simulink model "sampleModel7424_pp_1_1"  (R2018a)
settings: Solver=VariableStepAuto  StartTime=0.0  StopTime=10.0  RelTol=1e-3
undefined symbols (not defined in the file): DiscIntNeverNeededParam
libraries: simulink x211
(part 2 of 7)

== system sampleModel7424_pp_1_1/cfblk127 ==
  cfblk1 : Inport
  Action Port : ActionPort  ActionType=then
  cfblk10 : DiscreteFilter
  cfblk{5,7,9,11} (4 alike) : UnitDelay  SampleTime=-1
  cfblk12 : If  SampleTime=1
  cfblk18 : Subsystem  TreatAsAtomicUnit=on
  cfblk19 : Subsystem  TreatAsAtomicUnit=on
  cfblk20 : Delay
  cfblk21 : Delay
  cfblk3 : DiscreteIntegrator  SampleTime=-1  OutDataTypeStr=double  ICPrevOutput=DiscIntNeverNeededParam  ICPrevScaledInput=DiscIntNeverNeededParam
  cfblk4 : Delay
  cfblk6 : simulink/Continuous/PID Controller (2DOF)  Controller=PID  TimeDomain=Discrete-time  SampleTime=-1  IntegratorMethod=Forward Euler  FilterMethod=Forward Euler  Form=Parallel  UseFilter=on  ControllerParametersSource=internal  P=1  I=1  D=0  N=100  b=1  c=1  InitialConditionSource=internal  InitialConditionForIntegrator=0  InitialConditionForFilter=0  ExternalReset=none  LimitOutput=off  UpperSaturationLimit=inf  LowerSaturationLimit=-inf  LinearizeAsGain=off  AntiWindupMode=none  Kb=1  TrackingMode=off  Kt=1  PParamMin=[]  PParamMax=[]  IParamMin=[]  IParamMax=[]  DParamMin=[]  DParamMax=[]  NParamMin=[]  NParamMax=[]  bParamMin=[]  bParamMax=[]  cParamMin=[]  cParamMax=[]  KbParamMin=[]  KbParamMax=[]  KtParamMin=[]  KtParamMax=[]  POutMin=[]  POutMax=[]  IOutMin=[]  IOutMax=[]  DOutMin=[]  DOutMax=[]  NOutMin=[]  NOutMax=[]  bOutMin=[]  bOutMax=[]  cOutMin=[]  cOutMax=[]  KbOutMin=[]  KbOutMax=[]  KtOutMin=[]  KtOutMax=[]  IntegratorOutMin=[]  IntegratorOutMax=[]  FilterOutMin=[]  FilterOutMax=[]  SumOutMin=[]  SumOutMax=[]  Sum1OutMin=[]  Sum1OutMax=[]  Sum2OutMin=[]  Sum2OutMax=[]  Sum3OutMin=[]  Sum3OutMax=[]  SumI1OutMin=[]  SumI1OutMax=[]  SumI2OutMin=[]  SumI2OutMax=[]  SumI3OutMin=[]  SumI3OutMax=[]  SumDOutMin=[]  SumDOutMax=[]  SaturationOutMin=[]  SaturationOutMax=[]  IntegratorContinuousStateAttributes=''  IntegratorStateMustResolveToSignalObject=off  IntegratorRTWStateStorageClass=Auto  FilterContinuousStateAttributes=''  FilterStateMustResolveToSignalObject=off  FilterRTWStateStorageClass=Auto  DifferentiatorICPrevScaledInput=0  DifferentiatorOutMin=[]  DifferentiatorOutMax=[]  FilterDiffOutCoefMin=[]  FilterDiffOutCoefMax=[]  SumDenOutMin=[]  SumDenOutMax=[]  SumNumOutMin=[]  SumNumOutMax=[]  ReciprocalOutMin=[]  ReciprocalOutMax=[]  DivideOutMin=[]  DivideOutMax=[]  TunerSelectOption=Transfer Function Based (PID Tuner App)
  cfblk8 : simulink/Continuous/PID Controller  Controller=PID  TimeDomain=Discrete-time  SampleTime=-1  IntegratorMethod=Forward Euler  FilterMethod=Forward Euler  Form=Parallel  UseFilter=on  ControllerParametersSource=internal  P=1  I=1  D=0  N=100  InitialConditionSource=internal  InitialConditionForIntegrator=0  InitialConditionForFilter=0  ExternalReset=none  LimitOutput=off  UpperSaturationLimit=inf  LowerSaturationLimit=-inf  LinearizeAsGain=off  AntiWindupMode=none  Kb=1  TrackingMode=off  Kt=1  PParamMin=[]  PParamMax=[]  IParamMin=[]  IParamMax=[]  DParamMin=[]  DParamMax=[]  NParamMin=[]  NParamMax=[]  KbParamMin=[]  KbParamMax=[]  KtParamMin=[]  KtParamMax=[]  POutMin=[]  POutMax=[]  IOutMin=[]  IOutMax=[]  DOutMin=[]  DOutMax=[]  NOutMin=[]  NOutMax=[]  KbOutMin=[]  KbOutMax=[]  KtOutMin=[]  KtOutMax=[]  IntegratorOutMin=[]  IntegratorOutMax=[]  FilterOutMin=[]  FilterOutMax=[]  SumOutMin=[]  SumOutMax=[]  SumI1OutMin=[]  SumI1OutMax=[]  SumI2OutMin=[]  SumI2OutMax=[]  SumI3OutMin=[]  SumI3OutMax=[]  SumDOutMin=[]  SumDOutMax=[]  SaturationOutMin=[]  SaturationOutMax=[]  IntegratorContinuousStateAttributes=''  IntegratorStateMustResolveToSignalObject=off  IntegratorRTWStateStorageClass=Auto  FilterContinuousStateAttributes=''  FilterStateMustResolveToSignalObject=off  FilterRTWStateStorageClass=Auto  DifferentiatorICPrevScaledInput=0  DifferentiatorOutMin=[]  DifferentiatorOutMax=[]  FilterDiffOutCoefMin=[]  FilterDiffOutCoefMax=[]  SumDenOutMin=[]  SumDenOutMax=[]  SumNumOutMin=[]  SumNumOutMax=[]  ReciprocalOutMin=[]  ReciprocalOutMax=[]  DivideOutMin=[]  DivideOutMax=[]  TunerSelectOption=Transfer Function Based (PID Tuner App)
  cyemi_{227..230,239..240,253..262} (16 alike) : DataTypeConversion  OutDataTypeStr=double
  emi_{16,126,290,332} (4 alike) : UnaryMinus
  emi_127 : MATLAB Function  TreatAsAtomicUnit=on
  emi_17 : MATLAB Function  TreatAsAtomicUnit=on
  emi_291 : MATLAB Function  TreatAsAtomicUnit=on
  emi_333 : MATLAB Function  TreatAsAtomicUnit=on
  cfblk2 : Outport
  cfblk13 : Outport  Port=2
  cfblk14 : Outport  Port=3
  cfblk15 : Outport  Port=4
  cfblk16 : Outport  Port=5
  cfblk17 : Outport  Port=6
  wires:
  cfblk9/1 -> cfblk17/1
  cfblk8/1 -> cfblk2/1
  cfblk7/1 -> cyemi_253/1, cyemi_254/1
  cfblk19/1(cfblk2) -> cyemi_228/1, cyemi_257/1
  cfblk18/1(cfblk2) -> cyemi_255/1, cyemi_256/1
  cfblk10/1 -> cyemi_230/1, cyemi_258/1, cyemi_259/1
  cfblk6/1 -> cfblk16/1, cyemi_239/1, cyemi_261/1
  cfblk4/1 -> cfblk13/1
  cfblk1/1 -> cfblk14/1, cyemi_227/1
  cfblk3/1 -> cfblk15/1
  cfblk12/1 -> cfblk18/Action
  cfblk12/2 -> cfblk19/Action
  cyemi_227/1 -> cfblk10/1
  cyemi_228/1 -> cfblk11/1
  cyemi_229/1 -> cfblk12/1
  cfblk20/1 -> cyemi_229/1
  cyemi_230/1 -> cfblk18/1(cfblk1)
  cyemi_239/1 -> cfblk19/1(cfblk1)
  cyemi_240/1 -> cfblk19/2(cfblk10)
  cfblk21/1 -> cyemi_240/1
  cyemi_253/1 -> cfblk20/1, emi_126/1, emi_127/1(o)
  cyemi_254/1 -> cfblk21/1
  cyemi_255/1 -> cfblk3/1
  cyemi_256/1 -> cfblk4/1, emi_332/1, emi_333/1(o)
  cyemi_257/1 -> cfblk5/1, emi_290/1, emi_291/1(o)
  cyemi_258/1 -> cfblk6/1
  cyemi_259/1 -> cfblk6/2
  cyemi_260/1 -> cfblk7/1
  cfblk5/1 -> cyemi_260/1
  cyemi_261/1 -> cfblk8/1, emi_16/1, emi_17/1(o)
  cyemi_262/1 -> cfblk9/1
  cfblk11/1 -> cyemi_262/1
  emi_16/1 -> emi_17/2(e)
  emi_126/1 -> emi_127/2(e)
  emi_290/1 -> emi_291/2(e)
  emi_332/1 -> emi_333/2(e)

== system sampleModel7424_pp_1_1/cfblk128 ==
  cfblk1 : Inport
  cfblk9 : Inport  Port=2
  cfblk10 : Inport  Port=3
  Action Port : ActionPort  ActionType=else
  cfblk13 : DataTypeConversion  OutDataTypeStr=double
  cfblk14 : DataTypeConversion  OutDataTypeStr=double
  cfblk3 : simulink/Discrete/Transfer Fcn Lead or Lag  PoleZ=0.95  ZeroZ=0.75  ICPrevOutput=0.0  ICPrevInput=0.0  DoSatur=off
      settings: SourceProductName=Simulink  SourceProductBaseCode=SL
  cfblk4 : DiscreteIntegrator  SampleTime=-1  OutDataTypeStr=double  ICPrevOutput=DiscIntNeverNeededParam  ICPrevScaledInput=DiscIntNeverNeededParam
  cfblk5 : UnitDelay  SampleTime=-1
  cfblk6 : simulink/Discrete/Transfer Fcn First Order  PoleZ=0.95  ICPrevOutput=0.0  DoSatur=off
      settings: SourceProductName=Simulink
  cfblk7 : DiscreteStateSpace  SampleTime=-1
  cfblk8 : simulink/Discrete/Transfer Fcn Real Zero  ZeroZ=0.75  ICPrevInput=0.0  DoSatur=off
      settings: SourceProductName=Simulink  SourceProductBaseCode=SL
  cyemi_{266,269..270,272} (4 alike) : DataTypeConversion  OutDataTypeStr=double
  cyemi_267 : DataTypeConversion  OutDataTypeStr=fixdt('ufix16_E3')
  cyemi_268 : DataTypeConversion  OutDataTypeStr=uint16
  cyemi_271 : DataTypeConversion  OutDataTypeStr=fixdt('ufix16_E3')
  cyemi_273 : DataTypeConversion  OutDataTypeStr=fixdt('ufix16_E3')
  cfblk2 : Outport
  cfblk11 : Outport  Port=2
  cfblk12 : Outport  Port=3
  wires:
  cfblk5/1 -> cfblk11/1
  cfblk7/1 -> cfblk12/1
  cfblk10/1 -> cfblk2/1
  cyemi_266/1 -> cfblk13/1
  cfblk4/1 -> cyemi_266/1
  cyemi_267/1 -> cfblk14/1
  cfblk6/1 -> cyemi_267/1
  cyemi_268/1 -> cfblk3/1
  cfblk1/1 -> cyemi_268/1
  cyemi_269/1 -> cfblk4/1
  cfblk14/1 -> cyemi_269/1
  cyemi_270/1 -> cfblk5/1
  cfblk9/1 -> cyemi_270/1
  cyemi_271/1 -> cfblk6/1
  cfblk8/1 -> cyemi_271/1
  cyemi_272/1 -> cfblk7/1
  cfblk13/1 -> cyemi_272/1
  cyemi_273/1 -> cfblk8/1
  cfblk3/1 -> cyemi_273/1

== system sampleModel7424_pp_1_1/cfblk129 ==
  cfblk1 : Inport
  cfblk8 : Inport  Port=2
  Action Port : ActionPort  ActionType=then
  cfblk10 : Delay
  cfblk3 : UnitDelay  SampleTime=-1
  cfblk4 : simulink/Continuous/PID Controller (2DOF)  Controller=PID  TimeDomain=Discrete-time  SampleTime=-1  IntegratorMethod=Forward Euler  FilterMethod=Forward Euler  Form=Parallel  UseFilter=on  ControllerParametersSource=internal  P=1  I=1  D=0  N=100  b=1  c=1  InitialConditionSource=internal  InitialConditionForIntegrator=0  InitialConditionForFilter=0  ExternalReset=none  LimitOutput=off  UpperSaturationLimit=inf  LowerSaturationLimit=-inf  LinearizeAsGain=off  AntiWindupMode=none  Kb=1  TrackingMode=off  Kt=1  PParamMin=[]  PParamMax=[]  IParamMin=[]  IParamMax=[]  DParamMin=[]  DParamMax=[]  NParamMin=[]  NParamMax=[]  bParamMin=[]  bParamMax=[]  cParamMin=[]  cParamMax=[]  KbParamMin=[]  KbParamMax=[]  KtParamMin=[]  KtParamMax=[]  POutMin=[]  POutMax=[]  IOutMin=[]  IOutMax=[]  DOutMin=[]  DOutMax=[]  NOutMin=[]  NOutMax=[]  bOutMin=[]  bOutMax=[]  cOutMin=[]  cOutMax=[]  KbOutMin=[]  KbOutMax=[]  KtOutMin=[]  KtOutMax=[]  IntegratorOutMin=[]  IntegratorOutMax=[]  FilterOutMin=[]  FilterOutMax=[]  SumOutMin=[]  SumOutMax=[]  Sum1OutMin=[]  Sum1OutMax=[]  Sum2OutMin=[]  Sum2OutMax=[]  Sum3OutMin=[]  Sum3OutMax=[]  SumI1OutMin=[]  SumI1OutMax=[]  SumI2OutMin=[]  SumI2OutMax=[]  SumI3OutMin=[]  SumI3OutMax=[]  SumDOutMin=[]  SumDOutMax=[]  SaturationOutMin=[]  SaturationOutMax=[]  IntegratorContinuousStateAttributes=''  IntegratorStateMustResolveToSignalObject=off  IntegratorRTWStateStorageClass=Auto  FilterContinuousStateAttributes=''  FilterStateMustResolveToSignalObject=off  FilterRTWStateStorageClass=Auto  DifferentiatorICPrevScaledInput=0  DifferentiatorOutMin=[]  DifferentiatorOutMax=[]  FilterDiffOutCoefMin=[]  FilterDiffOutCoefMax=[]  SumDenOutMin=[]  SumDenOutMax=[]  SumNumOutMin=[]  SumNumOutMax=[]  ReciprocalOutMin=[]  ReciprocalOutMax=[]  DivideOutMin=[]  DivideOutMax=[]  TunerSelectOption=Transfer Function Based (PID Tuner App)
  cfblk5 : simulink/Continuous/PID Controller (2DOF)  Controller=PID  TimeDomain=Discrete-time  SampleTime=-1  IntegratorMethod=Forward Euler  FilterMethod=Forward Euler  Form=Parallel  UseFilter=on  ControllerParametersSource=internal  P=1  I=1  D=0  N=100  b=1  c=1  InitialConditionSource=internal  InitialConditionForIntegrator=0  InitialConditionForFilter=0  ExternalReset=none  LimitOutput=off  UpperSaturationLimit=inf  LowerSaturationLimit=-inf  LinearizeAsGain=off  AntiWindupMode=none  Kb=1  TrackingMode=off  Kt=1  PParamMin=[]  PParamMax=[]  IParamMin=[]  IParamMax=[]  DParamMin=[]  DParamMax=[]  NParamMin=[]  NParamMax=[]  bParamMin=[]  bParamMax=[]  cParamMin=[]  cParamMax=[]  KbParamMin=[]  KbParamMax=[]  KtParamMin=[]  KtParamMax=[]  POutMin=[]  POutMax=[]  IOutMin=[]  IOutMax=[]  DOutMin=[]  DOutMax=[]  NOutMin=[]  NOutMax=[]  bOutMin=[]  bOutMax=[]  cOutMin=[]  cOutMax=[]  KbOutMin=[]  KbOutMax=[]  KtOutMin=[]  KtOutMax=[]  IntegratorOutMin=[]  IntegratorOutMax=[]  FilterOutMin=[]  FilterOutMax=[]  SumOutMin=[]  SumOutMax=[]  Sum1OutMin=[]  Sum1OutMax=[]  Sum2OutMin=[]  Sum2OutMax=[]  Sum3OutMin=[]  Sum3OutMax=[]  SumI1OutMin=[]  SumI1OutMax=[]  SumI2OutMin=[]  SumI2OutMax=[]  SumI3OutMin=[]  SumI3OutMax=[]  SumDOutMin=[]  SumDOutMax=[]  SaturationOutMin=[]  SaturationOutMax=[]  IntegratorContinuousStateAttributes=''  IntegratorStateMustResolveToSignalObject=off  IntegratorRTWStateStorageClass=Auto  FilterContinuousStateAttributes=''  FilterStateMustResolveToSignalObject=off  FilterRTWStateStorageClass=Auto  DifferentiatorICPrevScaledInput=0  DifferentiatorOutMin=[]  DifferentiatorOutMax=[]  FilterDiffOutCoefMin=[]  FilterDiffOutCoefMax=[]  SumDenOutMin=[]  SumDenOutMax=[]  SumNumOutMin=[]  SumNumOutMax=[]  ReciprocalOutMin=[]  ReciprocalOutMax=[]  DivideOutMin=[]  DivideOutMax=[]  TunerSelectOption=Transfer Function Based (PID Tuner App)
  cfblk6 : UnitDelay  SampleTime=-1
  cfblk7 : simulink/Discrete/Transfer Fcn Lead or Lag  PoleZ=0.95  ZeroZ=0.75  ICPrevOutput=0.0  ICPrevInput=0.0  DoSatur=off
      settings: SourceProductName=Simulink  SourceProductBaseCode=SL
  cyemi_{276..283} (8 alike) : DataTypeConversion  OutDataTypeStr=double
  cfblk2 : Outport
  cfblk9 : Outport  Port=2
  wires:
  cfblk7/1 -> cfblk9/1
  cfblk8/1 -> cfblk2/1, cyemi_277/1, cyemi_281/1
  cyemi_276/1 -> cfblk10/1
  cfblk5/1 -> cyemi_276/1
  cyemi_277/1 -> cfblk3/1
  cyemi_278/1 -> cfblk4/1
  cfblk3/1 -> cyemi_278/1
  cyemi_279/1 -> cfblk4/2
  cfblk10/1 -> cyemi_279/1
  cyemi_280/1 -> cfblk5/1
  cfblk6/1 -> cyemi_280/1
  cyemi_281/1 -> cfblk5/2
  cyemi_282/1 -> cfblk6/1
  cfblk4/1 -> cyemi_282/1
  cyemi_283/1 -> cfblk7/1
  cfblk1/1 -> cyemi_283/1

== system sampleModel7424_pp_1_1/cfblk130 ==
  cfblk1 : Inport
  cfblk7 : Inport  Port=2
  cfblk8 : Inport  Port=3
  Action Port : ActionPort  ActionType=else
  cfblk11 : Subsystem  TreatAsAtomicUnit=on
  cfblk12 : Subsystem  TreatAsAtomicUnit=on
  cfblk13 : Delay
  cfblk14 : Delay
  cfblk3 : DiscreteFir
  cfblk4 : simulink/Continuous/PID Controller  Controller=PID  TimeDomain=Discrete-time  SampleTime=-1  IntegratorMethod=Forward Euler  FilterMethod=Forward Euler  Form=Parallel  UseFilter=on  ControllerParametersSource=internal  P=1  I=1  D=0  N=100  InitialConditionSource=internal  InitialConditionForIntegrator=0  InitialConditionForFilter=0  ExternalReset=none  LimitOutput=off  UpperSaturationLimit=inf  LowerSaturationLimit=-inf  LinearizeAsGain=off  AntiWindupMode=none  Kb=1  TrackingMode=off  Kt=1  PParamMin=[]  PParamMax=[]  IParamMin=[]  IParamMax=[]  DParamMin=[]  DParamMax=[]  NParamMin=[]  NParamMax=[]  KbParamMin=[]  KbParamMax=[]  KtParamMin=[]  KtParamMax=[]  POutMin=[]  POutMax=[]  IOutMin=[]  IOutMax=[]  DOutMin=[]  DOutMax=[]  NOutMin=[]  NOutMax=[]  KbOutMin=[]  KbOutMax=[]  KtOutMin=[]  KtOutMax=[]  IntegratorOutMin=[]  IntegratorOutMax=[]  FilterOutMin=[]  FilterOutMax=[]  SumOutMin=[]  SumOutMax=[]  SumI1OutMin=[]  SumI1OutMax=[]  SumI2OutMin=[]  SumI2OutMax=[]  SumI3OutMin=[]  SumI3OutMax=[]  SumDOutMin=[]  SumDOutMax=[]  SaturationOutMin=[]  SaturationOutMax=[]  IntegratorContinuousStateAttributes=''  IntegratorStateMustResolveToSignalObject=off  IntegratorRTWStateStorageClass=Auto  FilterContinuousStateAttributes=''  FilterStateMustResolveToSignalObject=off  FilterRTWStateStorageClass=Auto  DifferentiatorICPrevScaledInput=0  DifferentiatorOutMin=[]  DifferentiatorOutMax=[]  FilterDiffOutCoefMin=[]  FilterDiffOutCoefMax=[]  SumDenOutMin=[]  SumDenOutMax=[]  SumNumOutMin=[]  SumNumOutMax=[]  ReciprocalOutMin=[]  ReciprocalOutMax=[]  DivideOutMin=[]  DivideOutMax=[]  TunerSelectOption=Transfer Function Based (PID Tuner App)
  cfblk5 : UnitDelay  SampleTime=-1
  cfblk6 : If  SampleTime=1
  cyemi_{288..289,299..302,315..319} (11 alike) : DataTypeConversion  OutDataTypeStr=double
  cyemi_303 : DataTypeConversion  OutDataTypeStr=uint32
  cyemi_320 : DataTypeConversion  OutDataTypeStr=uint32
  emi_338 : UnaryMinus
  emi_339 : MATLAB Function  TreatAsAtomicUnit=on
  emi_50 : UnaryMinus
  emi_51 : MATLAB Function  TreatAsAtomicUnit=on
  cfblk2 : Outport
  cfblk9 : Outport  Port=2
  cfblk10 : Outport  Port=3
  wires:
  cfblk1/1 -> cyemi_288/1, cyemi_301/1
  cfblk11/2(cfblk10) -> cfblk2/1
  cfblk11/3(cfblk11) -> cfblk9/1, cyemi_302/1
  cfblk8/1 -> cyemi_303/1, cyemi_320/1
  cfblk12/1(cfblk2) -> cfblk10/1
  cfblk6/1 -> cfblk11/Action
  cfblk6/2 -> cfblk12/Action
  cyemi_288/1 -> cfblk11/1(cfblk1)
  cyemi_289/1 -> cfblk11/2(cfblk9)
  cfblk14/1 -> cyemi_289/1
  cyemi_299/1 -> cfblk12/1(cfblk1)
  cfblk13/1 -> cyemi_299/1
  cyemi_300/1 -> cfblk12/2(cfblk13)
  cfblk4/1 -> cyemi_300/1
  cyemi_301/1 -> cfblk12/3(cfblk14)
  cyemi_302/1 -> cfblk12/4(cfblk15)
  cyemi_303/1 -> cfblk12/5(cfblk16)
  cyemi_315/1 -> cfblk13/1, emi_338/1, emi_339/1(o)
  cfblk5/1 -> cyemi_315/1
  cyemi_316/1 -> cfblk14/1
  cfblk12/2(cfblk17) -> cyemi_316/1
  cyemi_317/1 -> cfblk3/1
  cfblk11/1(cfblk2) -> cyemi_317/1
  cyemi_318/1 -> cfblk4/1, emi_50/1, emi_51/1(o)
  cfblk7/1 -> cyemi_318/1
  cyemi_319/1 -> cfblk5/1
  cfblk3/1 -> cyemi_319/1
  cyemi_320/1 -> cfblk6/1
  emi_50/1 -> emi_51/2(e)
  emi_338/1 -> emi_339/2(e)

== system sampleModel7424_pp_1_1/cfblk131 ==
  cfblk1 : Inport
  cfblk13 : Inport  Port=2
  cfblk14 : Inport  Port=3
  Action Port : ActionPort  ActionType=then
  cfblk10 : simulink/Discrete/Transfer Fcn First Order  PoleZ=0.95  ICPrevOutput=0.0  DoSatur=off
      settings: SourceProductName=Simulink
  cfblk11 : simulink/Discrete/Difference  ICPrevInput=0.0  OutMin=[]  OutMax=[]  OutDataTypeStr=double  OutputDataTypeScalingMode=double  OutDataType=fixdt(1, 16)  OutScaling=2^-10  DoSatur=off
  cfblk12 : If  SampleTime=1
  cfblk16 : Subsystem  TreatAsAtomicUnit=on
  cfblk17 : Subsystem  TreatAsAtomicUnit=on
  cfblk{8,18..20} (4 alike) : Delay
  cfblk3 : simulink/Discrete/Tapped Delay  vinit=0.0  samptime=-1  NumDelays=1  DelayOrder=Oldest  includeCurrent=off
  cfblk4 : DiscreteStateSpace  SampleTime=-1
  cfblk5 : Delay  DelayLengthSource=Input port
      settings: InputPortMap=u0,p1
  cfblk6 : Delay  ShowEnablePort=on
      settings: InputPortMap=u0,e6
  cfblk7 : simulink/Discrete/Transfer Fcn First Order  PoleZ=0.95  ICPrevOutput=0.0  DoSatur=off
      settings: SourceProductName=Simulink
  cfblk9 : DiscreteIntegrator  SampleTime=-1  OutDataTypeStr=double  ICPrevOutput=DiscIntNeverNeededParam  ICPrevScaledInput=DiscIntNeverNeededParam
  cyemi_{324..328,340..341,347..358} (19 alike) : DataTypeConversion  OutDataTypeStr=double
  cfblk2 : Outport
  cfblk15 : Outport  Port=2
  wires:
  cfblk9/1 -> cfblk2/1, cyemi_354/1
  cfblk17/1(cfblk2) -> cyemi_325/1, cyemi_352/1
  cfblk8/1 -> cfblk15/1, cyemi_353/1
  cfblk12/1 -> cfblk16/Action
  cfblk12/2 -> cfblk17/Action
  cyemi_324/1 -> cfblk10/1
  cfblk16/2(cfblk13) -> cyemi_324/1
  cyemi_325/1 -> cfblk11/1
  cyemi_326/1 -> cfblk12/1
  cfblk14/1 -> cyemi_326/1
  cyemi_327/1 -> cfblk16/1(cfblk1)
  cfblk18/1 -> cyemi_327/1
  cyemi_328/1 -> cfblk16/2(cfblk12)
  cfblk3/1 -> cyemi_328/1
  cyemi_340/1 -> cfblk17/1(cfblk1)
  cfblk19/1 -> cyemi_340/1
  cyemi_341/1 -> cfblk17/2(cfblk8)
  cfblk20/1 -> cyemi_341/1
  cyemi_347/1 -> cfblk18/1
  cfblk5/1 -> cyemi_347/1
  cyemi_348/1 -> cfblk19/1
  cfblk4/1 -> cyemi_348/1
  cyemi_349/1 -> cfblk20/1
  cfblk11/1 -> cyemi_349/1
  cyemi_350/1 -> cfblk3/1
  cfblk1/1 -> cyemi_350/1
  cyemi_351/1 -> cfblk4/1
  cfblk10/1 -> cyemi_351/1
  cyemi_352/1 -> cfblk5/1
  cyemi_353/1 -> cfblk5/2
  cyemi_354/1 -> cfblk6/1
  cyemi_355/1 -> cfblk6/2
  cfblk7/1 -> cyemi_355/1
  cyemi_356/1 -> cfblk7/1
  cfblk13/1 -> cyemi_356/1
  cyemi_357/1 -> cfblk8/1
  cfblk6/1 -> cyemi_357/1
  cyemi_358/1 -> cfblk9/1
  cfblk16/1(cfblk2) -> cyemi_358/1

== system sampleModel7424_pp_1_1/cfblk132 ==
  cfblk1 : Inport
  cfblk13 : Inport  Port=2
  cfblk14 : Inport  Port=3
  Action Port : ActionPort  ActionType=else
  cfblk10 : simulink/Continuous/PID Controller (2DOF)  Controller=PID  TimeDomain=Discrete-time  SampleTime=-1  IntegratorMethod=Forward Euler  FilterMethod=Forward Euler  Form=Parallel  UseFilter=on  ControllerParametersSource=internal  P=1  I=1  D=0  N=100  b=1  c=1  InitialConditionSource=internal  InitialConditionForIntegrator=0  InitialConditionForFilter=0  ExternalReset=none  LimitOutput=off  UpperSaturationLimit=inf  LowerSaturationLimit=-inf  LinearizeAsGain=off  AntiWindupMode=none  Kb=1  TrackingMode=off  Kt=1  PParamMin=[]  PParamMax=[]  IParamMin=[]  IParamMax=[]  DParamMin=[]  DParamMax=[]  NParamMin=[]  NParamMax=[]  bParamMin=[]  bParamMax=[]  cParamMin=[]  cParamMax=[]  KbParamMin=[]  KbParamMax=[]  KtParamMin=[]  KtParamMax=[]  POutMin=[]  POutMax=[]  IOutMin=[]  IOutMax=[]  DOutMin=[]  DOutMax=[]  NOutMin=[]  NOutMax=[]  bOutMin=[]  bOutMax=[]  cOutMin=[]  cOutMax=[]  KbOutMin=[]  KbOutMax=[]  KtOutMin=[]  KtOutMax=[]  IntegratorOutMin=[]  IntegratorOutMax=[]  FilterOutMin=[]  FilterOutMax=[]  SumOutMin=[]  SumOutMax=[]  Sum1OutMin=[]  Sum1OutMax=[]  Sum2OutMin=[]  Sum2OutMax=[]  Sum3OutMin=[]  Sum3OutMax=[]  SumI1OutMin=[]  SumI1OutMax=[]  SumI2OutMin=[]  SumI2OutMax=[]  SumI3OutMin=[]  SumI3OutMax=[]  SumDOutMin=[]  SumDOutMax=[]  SaturationOutMin=[]  SaturationOutMax=[]  IntegratorContinuousStateAttributes=''  IntegratorStateMustResolveToSignalObject=off  IntegratorRTWStateStorageClass=Auto  FilterContinuousStateAttributes=''  FilterStateMustResolveToSignalObject=off  FilterRTWStateStorageClass=Auto  DifferentiatorICPrevScaledInput=0  DifferentiatorOutMin=[]  DifferentiatorOutMax=[]  FilterDiffOutCoefMin=[]  FilterDiffOutCoefMax=[]  SumDenOutMin=[]  SumDenOutMax=[]  SumNumOutMin=[]  SumNumOutMax=[]  ReciprocalOutMin=[]  ReciprocalOutMax=[]  DivideOutMin=[]  DivideOutMax=[]  TunerSelectOption=Transfer Function Based (PID Tuner App)
  cfblk11 : Delay
  cfblk12 : DiscreteFilter
  cfblk15 : Delay
  cfblk3 : simulink/Discrete/Transfer Fcn Real Zero  ZeroZ=0.75  ICPrevInput=0.0  DoSatur=off
      settings: SourceProductName=Simulink  SourceProductBaseCode=SL
  cfblk4 : DiscreteFir
  cfblk5 : DiscreteFilter
  cfblk6 : DiscreteIntegrator  SampleTime=-1  OutDataTypeStr=double  ICPrevOutput=DiscIntNeverNeededParam  ICPrevScaledInput=DiscIntNeverNeededParam
  cfblk7 : Delay  ShowEnablePort=on
      settings: InputPortMap=u0,e6
  cfblk8 : Delay  DelayLengthSource=Input port
      settings: InputPortMap=u0,p1
  cfblk9 : simulink/Discrete/Transfer Fcn First Order  PoleZ=0.95  ICPrevOutput=0.0  DoSatur=off
      settings: SourceProductName=Simulink
  cyemi_{362..363,365..375} (13 alike) : DataTypeConversion  OutDataTypeStr=double
  cyemi_364 : DataTypeConversion  OutDataTypeStr=uint16
  emi_{42,62,134,138,198} (5 alike) : UnaryMinus
  emi_135 : MATLAB Function  TreatAsAtomicUnit=on
  emi_139 : MATLAB Function  TreatAsAtomicUnit=on
  emi_199 : MATLAB Function  TreatAsAtomicUnit=on
  emi_43 : MATLAB Function  TreatAsAtomicUnit=on
  emi_63 : MATLAB Function  TreatAsAtomicUnit=on
  cfblk2 : Outport
  wires:
  cfblk13/1 -> cyemi_368/1, cyemi_375/1
  cfblk11/1 -> cfblk2/1
  cyemi_362/1 -> cfblk10/1, emi_198/1, emi_199/1(o)
  cfblk4/1 -> cyemi_362/1
  cyemi_363/1 -> cfblk10/2
  cfblk5/1 -> cyemi_363/1
  cyemi_364/1 -> cfblk11/1
  cfblk14/1 -> cyemi_364/1
  cyemi_365/1 -> cfblk12/1, emi_62/1, emi_63/1(o), emi_134/1, emi_135/1(o)
  cfblk6/1 -> cyemi_365/1
  cyemi_366/1 -> cfblk15/1, emi_138/1, emi_139/1(o)
  cfblk3/1 -> cyemi_366/1
  cyemi_367/1 -> cfblk3/1
  cfblk7/1 -> cyemi_367/1
  cyemi_368/1 -> cfblk4/1
  cyemi_369/1 -> cfblk5/1, emi_42/1, emi_43/1(o)
  cfblk1/1 -> cyemi_369/1
  cyemi_370/1 -> cfblk6/1
  cfblk9/1 -> cyemi_370/1
  cyemi_371/1 -> cfblk7/1
  cfblk8/1 -> cyemi_371/1
  cyemi_372/1 -> cfblk7/2
  cfblk12/1 -> cyemi_372/1
  cyemi_373/1 -> cfblk8/1
  cfblk15/1 -> cyemi_373/1
  cyemi_374/1 -> cfblk8/2
  cfblk10/1 -> cyemi_374/1
  cyemi_375/1 -> cfblk9/1
  emi_42/1 -> emi_43/2(e)
  emi_62/1 -> emi_63/2(e)
  emi_134/1 -> emi_135/2(e)
  emi_138/1 -> emi_139/2(e)
  emi_198/1 -> emi_199/2(e)

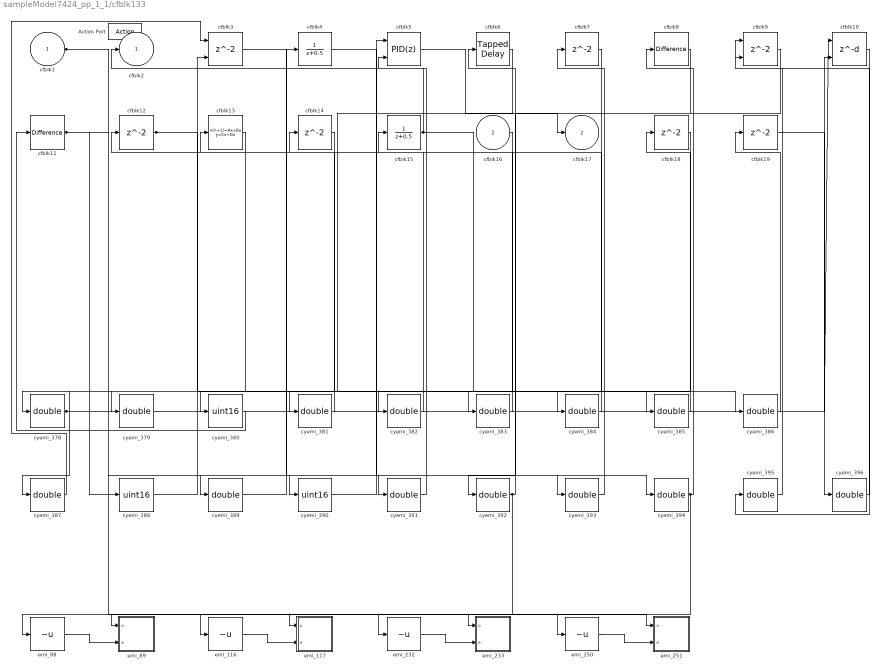
== system sampleModel7424_pp_1_1/cfblk133 ==
  cfblk1 : Inport
  cfblk16 : Inport  Port=2
  Action Port : ActionPort  ActionType=then
  cfblk10 : Delay  DelayLengthSource=Input port
      settings: InputPortMap=u0,p1
  cfblk11 : simulink/Discrete/Difference  ICPrevInput=0.0  OutMin=[]  OutMax=[]  OutDataTypeStr=uint16  OutputDataTypeScalingMode=uint16  OutDataType=fixdt(1, 16)  OutScaling=2^-10  DoSatur=off
  cfblk{7,12,14,18..19} (5 alike) : Delay
  cfblk13 : DiscreteStateSpace  SampleTime=-1
  cfblk15 : DiscreteTransferFcn
  cfblk3 : Delay  ShowEnablePort=on
      settings: InputPortMap=u0,e6
  cfblk4 : DiscreteTransferFcn
  cfblk5 : simulink/Continuous/PID Controller (2DOF)  Controller=PID  TimeDomain=Discrete-time  SampleTime=-1  IntegratorMethod=Forward Euler  FilterMethod=Forward Euler  Form=Parallel  UseFilter=on  ControllerParametersSource=internal  P=1  I=1  D=0  N=100  b=1  c=1  InitialConditionSource=internal  InitialConditionForIntegrator=0  InitialConditionForFilter=0  ExternalReset=none  LimitOutput=off  UpperSaturationLimit=inf  LowerSaturationLimit=-inf  LinearizeAsGain=off  AntiWindupMode=none  Kb=1  TrackingMode=off  Kt=1  PParamMin=[]  PParamMax=[]  IParamMin=[]  IParamMax=[]  DParamMin=[]  DParamMax=[]  NParamMin=[]  NParamMax=[]  bParamMin=[]  bParamMax=[]  cParamMin=[]  cParamMax=[]  KbParamMin=[]  KbParamMax=[]  KtParamMin=[]  KtParamMax=[]  POutMin=[]  POutMax=[]  IOutMin=[]  IOutMax=[]  DOutMin=[]  DOutMax=[]  NOutMin=[]  NOutMax=[]  bOutMin=[]  bOutMax=[]  cOutMin=[]  cOutMax=[]  KbOutMin=[]  KbOutMax=[]  KtOutMin=[]  KtOutMax=[]  IntegratorOutMin=[]  IntegratorOutMax=[]  FilterOutMin=[]  FilterOutMax=[]  SumOutMin=[]  SumOutMax=[]  Sum1OutMin=[]  Sum1OutMax=[]  Sum2OutMin=[]  Sum2OutMax=[]  Sum3OutMin=[]  Sum3OutMax=[]  SumI1OutMin=[]  SumI1OutMax=[]  SumI2OutMin=[]  SumI2OutMax=[]  SumI3OutMin=[]  SumI3OutMax=[]  SumDOutMin=[]  SumDOutMax=[]  SaturationOutMin=[]  SaturationOutMax=[]  IntegratorContinuousStateAttributes=''  IntegratorStateMustResolveToSignalObject=off  IntegratorRTWStateStorageClass=Auto  FilterContinuousStateAttributes=''  FilterStateMustResolveToSignalObject=off  FilterRTWStateStorageClass=Auto  DifferentiatorICPrevScaledInput=0  DifferentiatorOutMin=[]  DifferentiatorOutMax=[]  FilterDiffOutCoefMin=[]  FilterDiffOutCoefMax=[]  SumDenOutMin=[]  SumDenOutMax=[]  SumNumOutMin=[]  SumNumOutMax=[]  ReciprocalOutMin=[]  ReciprocalOutMax=[]  DivideOutMin=[]  DivideOutMax=[]  TunerSelectOption=Transfer Function Based (PID Tuner App)
  cfblk6 : simulink/Discrete/Tapped Delay  vinit=0.0  samptime=-1  NumDelays=1  DelayOrder=Oldest  includeCurrent=off
  cfblk8 : simulink/Discrete/Difference  ICPrevInput=0.0  OutMin=[]  OutMax=[]  OutDataTypeStr=double  OutputDataTypeScalingMode=double  OutDataType=fixdt(1, 16)  OutScaling=2^-10  DoSatur=off
  cfblk9 : Delay  ShowEnablePort=on
      settings: InputPortMap=u0,e6
  cyemi_{378..379,381..387,389,391..396} (16 alike) : DataTypeConversion  OutDataTypeStr=double
  cyemi_380 : DataTypeConversion  OutDataTypeStr=uint16
  cyemi_388 : DataTypeConversion  OutDataTypeStr=uint16
  cyemi_390 : DataTypeConversion  OutDataTypeStr=uint16
  emi_{88,116,232,250} (4 alike) : UnaryMinus
  emi_117 : MATLAB Function  TreatAsAtomicUnit=on
  emi_233 : MATLAB Function  TreatAsAtomicUnit=on
  emi_251 : MATLAB Function  TreatAsAtomicUnit=on
  emi_89 : MATLAB Function  TreatAsAtomicUnit=on
  cfblk2 : Outport
  cfblk17 : Outport  Port=2
  wires:
  cfblk15/1 -> cfblk2/1, cyemi_385/1
  cfblk12/1 -> cyemi_382/1, cyemi_386/1
  cfblk5/1 -> cfblk17/1
  cfblk11/1 -> cyemi_388/1, cyemi_390/1
  cfblk1/1 -> cyemi_389/1, cyemi_391/1
  cyemi_378/1 -> cfblk10/1, emi_250/1, emi_251/1(o)
  cfblk14/1 -> cyemi_378/1
  cyemi_379/1 -> cfblk10/2
  cfblk18/1 -> cyemi_379/1
  cyemi_380/1 -> cfblk11/1
  cfblk16/1 -> cyemi_380/1
  cyemi_381/1 -> cfblk12/1
  cfblk6/1 -> cyemi_381/1
  cyemi_382/1 -> cfblk13/1
  cyemi_383/1 -> cfblk14/1
  cfblk7/1 -> cyemi_383/1
  cyemi_384/1 -> cfblk15/1
  cfblk8/1 -> cyemi_384/1
  cyemi_385/1 -> cfblk18/1
  cyemi_386/1 -> cfblk19/1
  cyemi_387/1 -> cfblk3/1
  cfblk13/1 -> cyemi_387/1
  cyemi_388/1 -> cfblk3/2
  cyemi_389/1 -> cfblk4/1
  cyemi_390/1 -> cfblk5/1
  cyemi_391/1 -> cfblk5/2
  cyemi_392/1 -> cfblk6/1, emi_88/1, emi_89/1(o), emi_116/1, emi_117/1(o)
  cfblk9/1 -> cyemi_392/1
  cyemi_393/1 -> cfblk7/1
  cfblk4/1 -> cyemi_393/1
  cyemi_394/1 -> cfblk8/1, emi_232/1, emi_233/1(o)
  cfblk3/1 -> cyemi_394/1
  cyemi_395/1 -> cfblk9/1
  cfblk10/1 -> cyemi_395/1
  cyemi_396/1 -> cfblk9/2
  cfblk19/1 -> cyemi_396/1
  emi_88/1 -> emi_89/2(e)
  emi_116/1 -> emi_117/2(e)
  emi_232/1 -> emi_233/2(e)
  emi_250/1 -> emi_251/2(e)

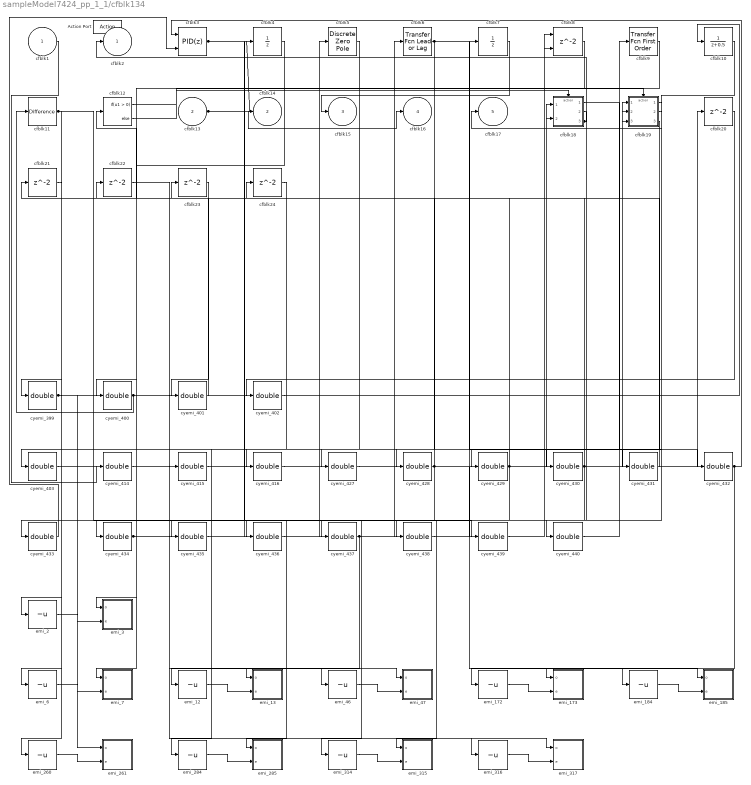
== system sampleModel7424_pp_1_1/cfblk134 ==
  cfblk1 : Inport
  cfblk13 : Inport  Port=2
  Action Port : ActionPort  ActionType=else
  cfblk10 : DiscreteTransferFcn
  cfblk11 : simulink/Discrete/Difference  ICPrevInput=0.0  OutMin=[]  OutMax=[]  OutDataTypeStr=double  OutputDataTypeScalingMode=double  OutDataType=fixdt(1, 16)  OutScaling=2^-10  DoSatur=off
  cfblk12 : If  SampleTime=1
  cfblk18 : Subsystem  TreatAsAtomicUnit=on
  cfblk19 : Subsystem  TreatAsAtomicUnit=on
  cfblk{20..24} (5 alike) : Delay
  cfblk3 : simulink/Continuous/PID Controller (2DOF)  Controller=PID  TimeDomain=Discrete-time  SampleTime=-1  IntegratorMethod=Forward Euler  FilterMethod=Forward Euler  Form=Parallel  UseFilter=on  ControllerParametersSource=internal  P=1  I=1  D=0  N=100  b=1  c=1  InitialConditionSource=internal  InitialConditionForIntegrator=0  InitialConditionForFilter=0  ExternalReset=none  LimitOutput=off  UpperSaturationLimit=inf  LowerSaturationLimit=-inf  LinearizeAsGain=off  AntiWindupMode=none  Kb=1  TrackingMode=off  Kt=1  PParamMin=[]  PParamMax=[]  IParamMin=[]  IParamMax=[]  DParamMin=[]  DParamMax=[]  NParamMin=[]  NParamMax=[]  bParamMin=[]  bParamMax=[]  cParamMin=[]  cParamMax=[]  KbParamMin=[]  KbParamMax=[]  KtParamMin=[]  KtParamMax=[]  POutMin=[]  POutMax=[]  IOutMin=[]  IOutMax=[]  DOutMin=[]  DOutMax=[]  NOutMin=[]  NOutMax=[]  bOutMin=[]  bOutMax=[]  cOutMin=[]  cOutMax=[]  KbOutMin=[]  KbOutMax=[]  KtOutMin=[]  KtOutMax=[]  IntegratorOutMin=[]  IntegratorOutMax=[]  FilterOutMin=[]  FilterOutMax=[]  SumOutMin=[]  SumOutMax=[]  Sum1OutMin=[]  Sum1OutMax=[]  Sum2OutMin=[]  Sum2OutMax=[]  Sum3OutMin=[]  Sum3OutMax=[]  SumI1OutMin=[]  SumI1OutMax=[]  SumI2OutMin=[]  SumI2OutMax=[]  SumI3OutMin=[]  SumI3OutMax=[]  SumDOutMin=[]  SumDOutMax=[]  SaturationOutMin=[]  SaturationOutMax=[]  IntegratorContinuousStateAttributes=''  IntegratorStateMustResolveToSignalObject=off  IntegratorRTWStateStorageClass=Auto  FilterContinuousStateAttributes=''  FilterStateMustResolveToSignalObject=off  FilterRTWStateStorageClass=Auto  DifferentiatorICPrevScaledInput=0  DifferentiatorOutMin=[]  DifferentiatorOutMax=[]  FilterDiffOutCoefMin=[]  FilterDiffOutCoefMax=[]  SumDenOutMin=[]  SumDenOutMax=[]  SumNumOutMin=[]  SumNumOutMax=[]  ReciprocalOutMin=[]  ReciprocalOutMax=[]  DivideOutMin=[]  DivideOutMax=[]  TunerSelectOption=Transfer Function Based (PID Tuner App)
  cfblk4 : UnitDelay  SampleTime=-1
  cfblk5 : DiscreteZeroPole  Poles=[0 0.5]  Gain=1  SampleTime=-1
  cfblk6 : simulink/Discrete/Transfer Fcn Lead or Lag  PoleZ=0.95  ZeroZ=0.75  ICPrevOutput=0.0  ICPrevInput=0.0  DoSatur=off
      settings: SourceProductName=Simulink  SourceProductBaseCode=SL
  cfblk7 : UnitDelay  SampleTime=-1
  cfblk8 : Delay  ShowEnablePort=on
      settings: InputPortMap=u0,e6
  cfblk9 : simulink/Discrete/Transfer Fcn First Order  PoleZ=0.95  ICPrevOutput=0.0  DoSatur=off
      settings: SourceProductName=Simulink
  cyemi_{399..403,414..416,427..440} (22 alike) : DataTypeConversion  OutDataTypeStr=double
  emi_{2,6,12,46,172,184,260,284,314,316} (10 alike) : UnaryMinus
  emi_13 : MATLAB Function  TreatAsAtomicUnit=on
  emi_173 : MATLAB Function  TreatAsAtomicUnit=on
  emi_185 : MATLAB Function  TreatAsAtomicUnit=on
  emi_261 : MATLAB Function  TreatAsAtomicUnit=on
  emi_285 : MATLAB Function  TreatAsAtomicUnit=on
  emi_3 : MATLAB Function  TreatAsAtomicUnit=on
  emi_315 : MATLAB Function  TreatAsAtomicUnit=on
  emi_317 : MATLAB Function  TreatAsAtomicUnit=on
  emi_47 : MATLAB Function  TreatAsAtomicUnit=on
  emi_7 : MATLAB Function  TreatAsAtomicUnit=on
  cfblk2 : Outport
  cfblk14 : Outport  Port=2
  cfblk15 : Outport  Port=3
  cfblk16 : Outport  Port=4
  cfblk17 : Outport  Port=5
  wires:
  cfblk7/1 -> cfblk15/1
  cfblk6/1 -> cyemi_427/1, cyemi_431/1
  cfblk13/1 -> cfblk16/1, cyemi_439/1
  cfblk3/1 -> cfblk14/1, cyemi_438/1
  cfblk11/1 -> cyemi_399/1, cyemi_437/1
  cfblk18/3(cfblk15) -> cfblk2/1, cyemi_440/1
  cfblk19/2(cfblk13) -> cfblk17/1
  cfblk12/1 -> cfblk18/Action
  cfblk12/2 -> cfblk19/Action
  cyemi_399/1 -> cfblk10/1, emi_260/1, emi_261/1(o)
  cyemi_400/1 -> cfblk11/1, emi_316/1, emi_317/1(o)
  cfblk4/1 -> cyemi_400/1
  cyemi_401/1 -> cfblk12/1
  cfblk23/1 -> cyemi_401/1
  cyemi_402/1 -> cfblk18/1(cfblk1)
  cfblk20/1 -> cyemi_402/1
  cyemi_403/1 -> cfblk18/2(cfblk13)
  cfblk21/1 -> cyemi_403/1
  cyemi_414/1 -> cfblk19/1(cfblk1)
  cfblk1/1 -> cyemi_414/1
  cyemi_415/1 -> cfblk19/2(cfblk11)
  cfblk22/1 -> cyemi_415/1
  cyemi_416/1 -> cfblk19/3(cfblk12)
  cfblk24/1 -> cyemi_416/1
  cyemi_427/1 -> cfblk20/1
  cyemi_428/1 -> cfblk21/1, emi_2/1, emi_3/1(o), emi_184/1, emi_185/1(o)
  cfblk8/1 -> cyemi_428/1
  cyemi_429/1 -> cfblk22/1, emi_6/1, emi_7/1(o)
  cfblk18/2(cfblk14) -> cyemi_429/1
  cyemi_430/1 -> cfblk23/1, emi_284/1, emi_285/1(o), emi_314/1, emi_315/1(o)
  cfblk10/1 -> cyemi_430/1
  cyemi_431/1 -> cfblk24/1
  cyemi_432/1 -> cfblk3/1, emi_172/1, emi_173/1(o)
  cfblk18/1(cfblk2) -> cyemi_432/1
  cyemi_433/1 -> cfblk3/2
  cfblk5/1 -> cyemi_433/1
  cyemi_434/1 -> cfblk4/1, emi_46/1, emi_47/1(o)
  cfblk9/1 -> cyemi_434/1
  cyemi_435/1 -> cfblk5/1
  cfblk19/3(cfblk14) -> cyemi_435/1
  cyemi_436/1 -> cfblk6/1
  cfblk19/1(cfblk2) -> cyemi_436/1
  cyemi_437/1 -> cfblk7/1, emi_12/1, emi_13/1(o)
  cyemi_438/1 -> cfblk8/1
  cyemi_439/1 -> cfblk8/2
  cyemi_440/1 -> cfblk9/1
  emi_2/1 -> emi_3/2(e)
  emi_6/1 -> emi_7/2(e)
  emi_12/1 -> emi_13/2(e)
  emi_46/1 -> emi_47/2(e)
  emi_172/1 -> emi_173/2(e)
  emi_184/1 -> emi_185/2(e)
  emi_260/1 -> emi_261/2(e)
  emi_284/1 -> emi_285/2(e)
  emi_314/1 -> emi_315/2(e)
  emi_316/1 -> emi_317/2(e)

== system sampleModel7424_pp_1_1/cfblk135 ==
  cfblk1 : Inport
  cfblk13 : Inport  Port=2
  Action Port : ActionPort  ActionType=then
  cfblk10 : simulink/Discrete/Transfer Fcn First Order  PoleZ=0.95  ICPrevOutput=0.0  DoSatur=off
      settings: SourceProductName=Simulink
  cfblk11 : simulink/Continuous/PID Controller (2DOF)  Controller=PID  TimeDomain=Discrete-time  SampleTime=-1  IntegratorMethod=Forward Euler  FilterMethod=Forward Euler  Form=Parallel  UseFilter=on  ControllerParametersSource=internal  P=1  I=1  D=0  N=100  b=1  c=1  InitialConditionSource=internal  InitialConditionForIntegrator=0  InitialConditionForFilter=0  ExternalReset=none  LimitOutput=off  UpperSaturationLimit=inf  LowerSaturationLimit=-inf  LinearizeAsGain=off  AntiWindupMode=none  Kb=1  TrackingMode=off  Kt=1  PParamMin=[]  PParamMax=[]  IParamMin=[]  IParamMax=[]  DParamMin=[]  DParamMax=[]  NParamMin=[]  NParamMax=[]  bParamMin=[]  bParamMax=[]  cParamMin=[]  cParamMax=[]  KbParamMin=[]  KbParamMax=[]  KtParamMin=[]  KtParamMax=[]  POutMin=[]  POutMax=[]  IOutMin=[]  IOutMax=[]  DOutMin=[]  DOutMax=[]  NOutMin=[]  NOutMax=[]  bOutMin=[]  bOutMax=[]  cOutMin=[]  cOutMax=[]  KbOutMin=[]  KbOutMax=[]  KtOutMin=[]  KtOutMax=[]  IntegratorOutMin=[]  IntegratorOutMax=[]  FilterOutMin=[]  FilterOutMax=[]  SumOutMin=[]  SumOutMax=[]  Sum1OutMin=[]  Sum1OutMax=[]  Sum2OutMin=[]  Sum2OutMax=[]  Sum3OutMin=[]  Sum3OutMax=[]  SumI1OutMin=[]  SumI1OutMax=[]  SumI2OutMin=[]  SumI2OutMax=[]  SumI3OutMin=[]  SumI3OutMax=[]  SumDOutMin=[]  SumDOutMax=[]  SaturationOutMin=[]  SaturationOutMax=[]  IntegratorContinuousStateAttributes=''  IntegratorStateMustResolveToSignalObject=off  IntegratorRTWStateStorageClass=Auto  FilterContinuousStateAttributes=''  FilterStateMustResolveToSignalObject=off  FilterRTWStateStorageClass=Auto  DifferentiatorICPrevScaledInput=0  DifferentiatorOutMin=[]  DifferentiatorOutMax=[]  FilterDiffOutCoefMin=[]  FilterDiffOutCoefMax=[]  SumDenOutMin=[]  SumDenOutMax=[]  SumNumOutMin=[]  SumNumOutMax=[]  ReciprocalOutMin=[]  ReciprocalOutMax=[]  DivideOutMin=[]  DivideOutMax=[]  TunerSelectOption=Transfer Function Based (PID Tuner App)
  cfblk12 : UnitDelay  SampleTime=-1
  cfblk15 : Delay
  cfblk16 : Delay
  cfblk3 : simulink/Continuous/PID Controller (2DOF)  Controller=PID  TimeDomain=Discrete-time  SampleTime=-1  IntegratorMethod=Forward Euler  FilterMethod=Forward Euler  Form=Parallel  UseFilter=on  ControllerParametersSource=internal  P=1  I=1  D=0  N=100  b=1  c=1  InitialConditionSource=internal  InitialConditionForIntegrator=0  InitialConditionForFilter=0  ExternalReset=none  LimitOutput=off  UpperSaturationLimit=inf  LowerSaturationLimit=-inf  LinearizeAsGain=off  AntiWindupMode=none  Kb=1  TrackingMode=off  Kt=1  PParamMin=[]  PParamMax=[]  IParamMin=[]  IParamMax=[]  DParamMin=[]  DParamMax=[]  NParamMin=[]  NParamMax=[]  bParamMin=[]  bParamMax=[]  cParamMin=[]  cParamMax=[]  KbParamMin=[]  KbParamMax=[]  KtParamMin=[]  KtParamMax=[]  POutMin=[]  POutMax=[]  IOutMin=[]  IOutMax=[]  DOutMin=[]  DOutMax=[]  NOutMin=[]  NOutMax=[]  bOutMin=[]  bOutMax=[]  cOutMin=[]  cOutMax=[]  KbOutMin=[]  KbOutMax=[]  KtOutMin=[]  KtOutMax=[]  IntegratorOutMin=[]  IntegratorOutMax=[]  FilterOutMin=[]  FilterOutMax=[]  SumOutMin=[]  SumOutMax=[]  Sum1OutMin=[]  Sum1OutMax=[]  Sum2OutMin=[]  Sum2OutMax=[]  Sum3OutMin=[]  Sum3OutMax=[]  SumI1OutMin=[]  SumI1OutMax=[]  SumI2OutMin=[]  SumI2OutMax=[]  SumI3OutMin=[]  SumI3OutMax=[]  SumDOutMin=[]  SumDOutMax=[]  SaturationOutMin=[]  SaturationOutMax=[]  IntegratorContinuousStateAttributes=''  IntegratorStateMustResolveToSignalObject=off  IntegratorRTWStateStorageClass=Auto  FilterContinuousStateAttributes=''  FilterStateMustResolveToSignalObject=off  FilterRTWStateStorageClass=Auto  DifferentiatorICPrevScaledInput=0  DifferentiatorOutMin=[]  DifferentiatorOutMax=[]  FilterDiffOutCoefMin=[]  FilterDiffOutCoefMax=[]  SumDenOutMin=[]  SumDenOutMax=[]  SumNumOutMin=[]  SumNumOutMax=[]  ReciprocalOutMin=[]  ReciprocalOutMax=[]  DivideOutMin=[]  DivideOutMax=[]  TunerSelectOption=Transfer Function Based (PID Tuner App)
  cfblk4 : DiscreteZeroPole  Poles=[0 0.5]  Gain=1  SampleTime=-1
  cfblk5 : DiscreteIntegrator  SampleTime=-1  OutDataTypeStr=double  ICPrevOutput=DiscIntNeverNeededParam  ICPrevScaledInput=DiscIntNeverNeededParam
  cfblk6 : simulink/Discrete/Transfer Fcn Lead or Lag  PoleZ=0.95  ZeroZ=0.75  ICPrevOutput=0.0  ICPrevInput=0.0  DoSatur=off
      settings: SourceProductName=Simulink  SourceProductBaseCode=SL
  cfblk7 : Delay  DelayLengthSource=Input port
      settings: InputPortMap=u0,p1
  cfblk8 : DiscreteFilter
  cfblk9 : simulink/Continuous/PID Controller  Controller=PID  TimeDomain=Discrete-time  SampleTime=-1  IntegratorMethod=Forward Euler  FilterMethod=Forward Euler  Form=Parallel  UseFilter=on  ControllerParametersSource=internal  P=1  I=1  D=0  N=100  InitialConditionSource=internal  InitialConditionForIntegrator=0  InitialConditionForFilter=0  ExternalReset=none  LimitOutput=off  UpperSaturationLimit=inf  LowerSaturationLimit=-inf  LinearizeAsGain=off  AntiWindupMode=none  Kb=1  TrackingMode=off  Kt=1  PParamMin=[]  PParamMax=[]  IParamMin=[]  IParamMax=[]  DParamMin=[]  DParamMax=[]  NParamMin=[]  NParamMax=[]  KbParamMin=[]  KbParamMax=[]  KtParamMin=[]  KtParamMax=[]  POutMin=[]  POutMax=[]  IOutMin=[]  IOutMax=[]  DOutMin=[]  DOutMax=[]  NOutMin=[]  NOutMax=[]  KbOutMin=[]  KbOutMax=[]  KtOutMin=[]  KtOutMax=[]  IntegratorOutMin=[]  IntegratorOutMax=[]  FilterOutMin=[]  FilterOutMax=[]  SumOutMin=[]  SumOutMax=[]  SumI1OutMin=[]  SumI1OutMax=[]  SumI2OutMin=[]  SumI2OutMax=[]  SumI3OutMin=[]  SumI3OutMax=[]  SumDOutMin=[]  SumDOutMax=[]  SaturationOutMin=[]  SaturationOutMax=[]  IntegratorContinuousStateAttributes=''  IntegratorStateMustResolveToSignalObject=off  IntegratorRTWStateStorageClass=Auto  FilterContinuousStateAttributes=''  FilterStateMustResolveToSignalObject=off  FilterRTWStateStorageClass=Auto  DifferentiatorICPrevScaledInput=0  DifferentiatorOutMin=[]  DifferentiatorOutMax=[]  FilterDiffOutCoefMin=[]  FilterDiffOutCoefMax=[]  SumDenOutMin=[]  SumDenOutMax=[]  SumNumOutMin=[]  SumNumOutMax=[]  ReciprocalOutMin=[]  ReciprocalOutMax=[]  DivideOutMin=[]  DivideOutMax=[]  TunerSelectOption=Transfer Function Based (PID Tuner App)
  cyemi_{443..457} (15 alike) : DataTypeConversion  OutDataTypeStr=double
  cfblk2 : Outport
  cfblk14 : Outport  Port=2
  wires:
  cfblk11/1 -> cyemi_451/1, cyemi_452/1
  cfblk8/1 -> cfblk14/1, cyemi_448/1
  cfblk6/1 -> cyemi_445/1, cyemi_454/1
  cfblk4/1 -> cfblk2/1
  cyemi_443/1 -> cfblk10/1
  cfblk1/1 -> cyemi_443/1
  cyemi_444/1 -> cfblk11/1
  cfblk12/1 -> cyemi_444/1
  cyemi_445/1 -> cfblk11/2
  cyemi_446/1 -> cfblk12/1
  cfblk13/1 -> cyemi_446/1
  cyemi_447/1 -> cfblk15/1
  cfblk9/1 -> cyemi_447/1
  cyemi_448/1 -> cfblk16/1
  cyemi_449/1 -> cfblk3/1
  cfblk5/1 -> cyemi_449/1
  cyemi_450/1 -> cfblk3/2
  cfblk16/1 -> cyemi_450/1
  cyemi_451/1 -> cfblk4/1
  cyemi_452/1 -> cfblk5/1
  cyemi_453/1 -> cfblk6/1
  cfblk10/1 -> cyemi_453/1
  cyemi_454/1 -> cfblk7/1
  cyemi_455/1 -> cfblk7/2
  cfblk15/1 -> cyemi_455/1
  cyemi_456/1 -> cfblk8/1
  cfblk3/1 -> cyemi_456/1
  cyemi_457/1 -> cfblk9/1
  cfblk7/1 -> cyemi_457/1

== system sampleModel7424_pp_1_1/cfblk136 ==
  cfblk1 : Inport
  Action Port : ActionPort  ActionType=else
  cfblk10 : simulink/Discrete/Difference  ICPrevInput=0.0  OutMin=[]  OutMax=[]  OutDataTypeStr=double  OutputDataTypeScalingMode=double  OutDataType=fixdt(1, 16)  OutScaling=2^-10  DoSatur=off
  cfblk11 : Delay
  cfblk12 : Delay
  cfblk3 : simulink/Continuous/PID Controller (2DOF)  Controller=PID  TimeDomain=Discrete-time  SampleTime=-1  IntegratorMethod=Forward Euler  FilterMethod=Forward Euler  Form=Parallel  UseFilter=on  ControllerParametersSource=internal  P=1  I=1  D=0  N=100  b=1  c=1  InitialConditionSource=internal  InitialConditionForIntegrator=0  InitialConditionForFilter=0  ExternalReset=none  LimitOutput=off  UpperSaturationLimit=inf  LowerSaturationLimit=-inf  LinearizeAsGain=off  AntiWindupMode=none  Kb=1  TrackingMode=off  Kt=1  PParamMin=[]  PParamMax=[]  IParamMin=[]  IParamMax=[]  DParamMin=[]  DParamMax=[]  NParamMin=[]  NParamMax=[]  bParamMin=[]  bParamMax=[]  cParamMin=[]  cParamMax=[]  KbParamMin=[]  KbParamMax=[]  KtParamMin=[]  KtParamMax=[]  POutMin=[]  POutMax=[]  IOutMin=[]  IOutMax=[]  DOutMin=[]  DOutMax=[]  NOutMin=[]  NOutMax=[]  bOutMin=[]  bOutMax=[]  cOutMin=[]  cOutMax=[]  KbOutMin=[]  KbOutMax=[]  KtOutMin=[]  KtOutMax=[]  IntegratorOutMin=[]  IntegratorOutMax=[]  FilterOutMin=[]  FilterOutMax=[]  SumOutMin=[]  SumOutMax=[]  Sum1OutMin=[]  Sum1OutMax=[]  Sum2OutMin=[]  Sum2OutMax=[]  Sum3OutMin=[]  Sum3OutMax=[]  SumI1OutMin=[]  SumI1OutMax=[]  SumI2OutMin=[]  SumI2OutMax=[]  SumI3OutMin=[]  SumI3OutMax=[]  SumDOutMin=[]  SumDOutMax=[]  SaturationOutMin=[]  SaturationOutMax=[]  IntegratorContinuousStateAttributes=''  IntegratorStateMustResolveToSignalObject=off  IntegratorRTWStateStorageClass=Auto  FilterContinuousStateAttributes=''  FilterStateMustResolveToSignalObject=off  FilterRTWStateStorageClass=Auto  DifferentiatorICPrevScaledInput=0  DifferentiatorOutMin=[]  DifferentiatorOutMax=[]  FilterDiffOutCoefMin=[]  FilterDiffOutCoefMax=[]  SumDenOutMin=[]  SumDenOutMax=[]  SumNumOutMin=[]  SumNumOutMax=[]  ReciprocalOutMin=[]  ReciprocalOutMax=[]  DivideOutMin=[]  DivideOutMax=[]  TunerSelectOption=Transfer Function Based (PID Tuner App)
  cfblk4 : simulink/Continuous/PID Controller  Controller=PID  TimeDomain=Discrete-time  SampleTime=-1  IntegratorMethod=Forward Euler  FilterMethod=Forward Euler  Form=Parallel  UseFilter=on  ControllerParametersSource=internal  P=1  I=1  D=0  N=100  InitialConditionSource=internal  InitialConditionForIntegrator=0  InitialConditionForFilter=0  ExternalReset=none  LimitOutput=off  UpperSaturationLimit=inf  LowerSaturationLimit=-inf  LinearizeAsGain=off  AntiWindupMode=none  Kb=1  TrackingMode=off  Kt=1  PParamMin=[]  PParamMax=[]  IParamMin=[]  IParamMax=[]  DParamMin=[]  DParamMax=[]  NParamMin=[]  NParamMax=[]  KbParamMin=[]  KbParamMax=[]  KtParamMin=[]  KtParamMax=[]  POutMin=[]  POutMax=[]  IOutMin=[]  IOutMax=[]  DOutMin=[]  DOutMax=[]  NOutMin=[]  NOutMax=[]  KbOutMin=[]  KbOutMax=[]  KtOutMin=[]  KtOutMax=[]  IntegratorOutMin=[]  IntegratorOutMax=[]  FilterOutMin=[]  FilterOutMax=[]  SumOutMin=[]  SumOutMax=[]  SumI1OutMin=[]  SumI1OutMax=[]  SumI2OutMin=[]  SumI2OutMax=[]  SumI3OutMin=[]  SumI3OutMax=[]  SumDOutMin=[]  SumDOutMax=[]  SaturationOutMin=[]  SaturationOutMax=[]  IntegratorContinuousStateAttributes=''  IntegratorStateMustResolveToSignalObject=off  IntegratorRTWStateStorageClass=Auto  FilterContinuousStateAttributes=''  FilterStateMustResolveToSignalObject=off  FilterRTWStateStorageClass=Auto  DifferentiatorICPrevScaledInput=0  DifferentiatorOutMin=[]  DifferentiatorOutMax=[]  FilterDiffOutCoefMin=[]  FilterDiffOutCoefMax=[]  SumDenOutMin=[]  SumDenOutMax=[]  SumNumOutMin=[]  SumNumOutMax=[]  ReciprocalOutMin=[]  ReciprocalOutMax=[]  DivideOutMin=[]  DivideOutMax=[]  TunerSelectOption=Transfer Function Based (PID Tuner App)
  cfblk5 : simulink/Continuous/PID Controller (2DOF)  Controller=PID  TimeDomain=Discrete-time  SampleTime=-1  IntegratorMethod=Forward Euler  FilterMethod=Forward Euler  Form=Parallel  UseFilter=on  ControllerParametersSource=internal  P=1  I=1  D=0  N=100  b=1  c=1  InitialConditionSource=internal  InitialConditionForIntegrator=0  InitialConditionForFilter=0  ExternalReset=none  LimitOutput=off  UpperSaturationLimit=inf  LowerSaturationLimit=-inf  LinearizeAsGain=off  AntiWindupMode=none  Kb=1  TrackingMode=off  Kt=1  PParamMin=[]  PParamMax=[]  IParamMin=[]  IParamMax=[]  DParamMin=[]  DParamMax=[]  NParamMin=[]  NParamMax=[]  bParamMin=[]  bParamMax=[]  cParamMin=[]  cParamMax=[]  KbParamMin=[]  KbParamMax=[]  KtParamMin=[]  KtParamMax=[]  POutMin=[]  POutMax=[]  IOutMin=[]  IOutMax=[]  DOutMin=[]  DOutMax=[]  NOutMin=[]  NOutMax=[]  bOutMin=[]  bOutMax=[]  cOutMin=[]  cOutMax=[]  KbOutMin=[]  KbOutMax=[]  KtOutMin=[]  KtOutMax=[]  IntegratorOutMin=[]  IntegratorOutMax=[]  FilterOutMin=[]  FilterOutMax=[]  SumOutMin=[]  SumOutMax=[]  Sum1OutMin=[]  Sum1OutMax=[]  Sum2OutMin=[]  Sum2OutMax=[]  Sum3OutMin=[]  Sum3OutMax=[]  SumI1OutMin=[]  SumI1OutMax=[]  SumI2OutMin=[]  SumI2OutMax=[]  SumI3OutMin=[]  SumI3OutMax=[]  SumDOutMin=[]  SumDOutMax=[]  SaturationOutMin=[]  SaturationOutMax=[]  IntegratorContinuousStateAttributes=''  IntegratorStateMustResolveToSignalObject=off  IntegratorRTWStateStorageClass=Auto  FilterContinuousStateAttributes=''  FilterStateMustResolveToSignalObject=off  FilterRTWStateStorageClass=Auto  DifferentiatorICPrevScaledInput=0  DifferentiatorOutMin=[]  DifferentiatorOutMax=[]  FilterDiffOutCoefMin=[]  FilterDiffOutCoefMax=[]  SumDenOutMin=[]  SumDenOutMax=[]  SumNumOutMin=[]  SumNumOutMax=[]  ReciprocalOutMin=[]  ReciprocalOutMax=[]  DivideOutMin=[]  DivideOutMax=[]  TunerSelectOption=Transfer Function Based (PID Tuner App)
  cfblk6 : simulink/Discrete/Transfer Fcn First Order  PoleZ=0.95  ICPrevOutput=0.0  DoSatur=off
      settings: SourceProductName=Simulink
  cfblk7 : simulink/Continuous/PID Controller  Controller=PID  TimeDomain=Discrete-time  SampleTime=-1  IntegratorMethod=Forward Euler  FilterMethod=Forward Euler  Form=Parallel  UseFilter=on  ControllerParametersSource=internal  P=1  I=1  D=0  N=100  InitialConditionSource=internal  InitialConditionForIntegrator=0  InitialConditionForFilter=0  ExternalReset=none  LimitOutput=off  UpperSaturationLimit=inf  LowerSaturationLimit=-inf  LinearizeAsGain=off  AntiWindupMode=none  Kb=1  TrackingMode=off  Kt=1  PParamMin=[]  PParamMax=[]  IParamMin=[]  IParamMax=[]  DParamMin=[]  DParamMax=[]  NParamMin=[]  NParamMax=[]  KbParamMin=[]  KbParamMax=[]  KtParamMin=[]  KtParamMax=[]  POutMin=[]  POutMax=[]  IOutMin=[]  IOutMax=[]  DOutMin=[]  DOutMax=[]  NOutMin=[]  NOutMax=[]  KbOutMin=[]  KbOutMax=[]  KtOutMin=[]  KtOutMax=[]  IntegratorOutMin=[]  IntegratorOutMax=[]  FilterOutMin=[]  FilterOutMax=[]  SumOutMin=[]  SumOutMax=[]  SumI1OutMin=[]  SumI1OutMax=[]  SumI2OutMin=[]  SumI2OutMax=[]  SumI3OutMin=[]  SumI3OutMax=[]  SumDOutMin=[]  SumDOutMax=[]  SaturationOutMin=[]  SaturationOutMax=[]  IntegratorContinuousStateAttributes=''  IntegratorStateMustResolveToSignalObject=off  IntegratorRTWStateStorageClass=Auto  FilterContinuousStateAttributes=''  FilterStateMustResolveToSignalObject=off  FilterRTWStateStorageClass=Auto  DifferentiatorICPrevScaledInput=0  DifferentiatorOutMin=[]  DifferentiatorOutMax=[]  FilterDiffOutCoefMin=[]  FilterDiffOutCoefMax=[]  SumDenOutMin=[]  SumDenOutMax=[]  SumNumOutMin=[]  SumNumOutMax=[]  ReciprocalOutMin=[]  ReciprocalOutMax=[]  DivideOutMin=[]  DivideOutMax=[]  TunerSelectOption=Transfer Function Based (PID Tuner App)
  cfblk8 : Delay
  cfblk9 : Delay  DelayLengthSource=Input port
      settings: InputPortMap=u0,p1
  cyemi_{459..471} (13 alike) : DataTypeConversion  OutDataTypeStr=double
  emi_{40,84,182,226,310} (5 alike) : UnaryMinus
  emi_183 : MATLAB Function  TreatAsAtomicUnit=on
  emi_227 : MATLAB Function  TreatAsAtomicUnit=on
  emi_311 : MATLAB Function  TreatAsAtomicUnit=on
  emi_41 : MATLAB Function  TreatAsAtomicUnit=on
  emi_85 : MATLAB Function  TreatAsAtomicUnit=on
  cfblk2 : Outport
  wires:
  cfblk1/1 -> cyemi_467/1, cyemi_470/1
  cfblk8/1 -> cyemi_459/1, cyemi_465/1
  cfblk4/1 -> cyemi_460/1, cyemi_466/1
  cfblk6/1 -> cfblk2/1
  cyemi_459/1 -> cfblk10/1
  cyemi_460/1 -> cfblk11/1
  cyemi_461/1 -> cfblk12/1
  cfblk5/1 -> cyemi_461/1
  cyemi_462/1 -> cfblk3/1, emi_310/1, emi_311/1(o)
  cfblk12/1 -> cyemi_462/1
  cyemi_463/1 -> cfblk3/2
  cfblk7/1 -> cyemi_463/1
  cyemi_464/1 -> cfblk4/1
  cfblk10/1 -> cyemi_464/1
  cyemi_465/1 -> cfblk5/1, emi_40/1, emi_41/1(o), emi_84/1, emi_85/1(o), emi_226/1, emi_227/1(o)
  cyemi_466/1 -> cfblk5/2
  cyemi_467/1 -> cfblk6/1
  cyemi_468/1 -> cfblk7/1
  cfblk9/1 -> cyemi_468/1
  cyemi_469/1 -> cfblk8/1
  cfblk3/1 -> cyemi_469/1
  cyemi_470/1 -> cfblk9/1, emi_182/1, emi_183/1(o)
  cyemi_471/1 -> cfblk9/2
  cfblk11/1 -> cyemi_471/1
  emi_40/1 -> emi_41/2(e)
  emi_84/1 -> emi_85/2(e)
  emi_182/1 -> emi_183/2(e)
  emi_226/1 -> emi_227/2(e)
  emi_310/1 -> emi_311/2(e)
